simulink model "RefuelSystem"  (R2025a)
settings: Solver=ode23tb  StartTime=0.0  StopTime=1000  MaxStep=0.1  RelTol=1e-3
libraries: simulink x5
settings Model: DataDictionary=FuelGaugingData.sldd  Creator=mkelley  LastModifiedBy=mkelley

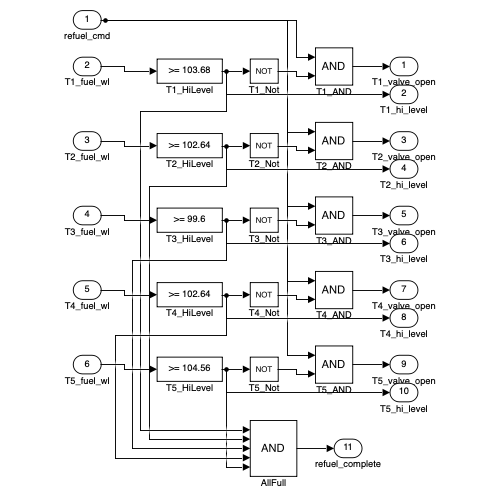
[thumbnail: Simulink's stored preview of the top-level diagram]
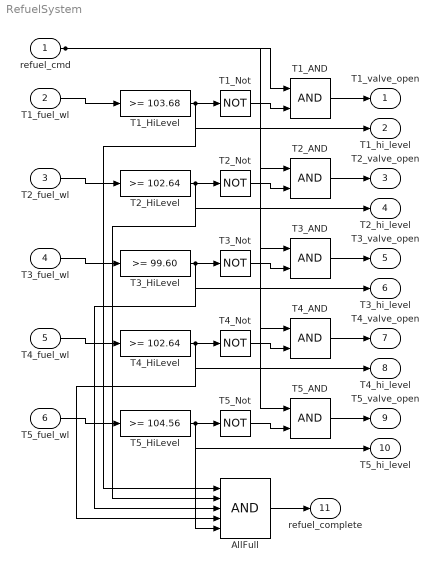
== system RefuelSystem ==
  refuel_cmd : Inport
  T1_fuel_wl : Inport  Port=2
  T2_fuel_wl : Inport  Port=3
  T3_fuel_wl : Inport  Port=4
  T4_fuel_wl : Inport  Port=5
  T5_fuel_wl : Inport  Port=6
  AllFull : Logic  Inputs=5  AllPortsSameDT=off  OutDataTypeStr=boolean
  T1_AND : Logic  AllPortsSameDT=off  OutDataTypeStr=boolean
  T1_HiLevel : simulink/Logic and Bit Operations/Compare To Constant  relop=>=  const=103.68  OutDataTypeStr=boolean
  T1_Not : Logic  Operator=NOT  AllPortsSameDT=off  OutDataTypeStr=boolean
  T2_AND : Logic  AllPortsSameDT=off  OutDataTypeStr=boolean
  T2_HiLevel : simulink/Logic and Bit Operations/Compare To Constant  relop=>=  const=102.64  OutDataTypeStr=boolean
  T2_Not : Logic  Operator=NOT  AllPortsSameDT=off  OutDataTypeStr=boolean
  T3_AND : Logic  AllPortsSameDT=off  OutDataTypeStr=boolean
  T3_HiLevel : simulink/Logic and Bit Operations/Compare To Constant  relop=>=  const=99.60  OutDataTypeStr=boolean
  T3_Not : Logic  Operator=NOT  AllPortsSameDT=off  OutDataTypeStr=boolean
  T4_AND : Logic  AllPortsSameDT=off  OutDataTypeStr=boolean
  T4_HiLevel : simulink/Logic and Bit Operations/Compare To Constant  relop=>=  const=102.64  OutDataTypeStr=boolean
  T4_Not : Logic  Operator=NOT  AllPortsSameDT=off  OutDataTypeStr=boolean
  T5_AND : Logic  AllPortsSameDT=off  OutDataTypeStr=boolean
  T5_HiLevel : simulink/Logic and Bit Operations/Compare To Constant  relop=>=  const=104.56  OutDataTypeStr=boolean
  T5_Not : Logic  Operator=NOT  AllPortsSameDT=off  OutDataTypeStr=boolean
  T1_valve_open : Outport
  T1_hi_level : Outport  Port=2
  T2_valve_open : Outport  Port=3
  T2_hi_level : Outport  Port=4
  T3_valve_open : Outport  Port=5
  T3_hi_level : Outport  Port=6
  T4_valve_open : Outport  Port=7
  T4_hi_level : Outport  Port=8
  T5_valve_open : Outport  Port=9
  T5_hi_level : Outport  Port=10
  refuel_complete : Outport  Port=11
  wires:
  T1_fuel_wl/1 -> T1_HiLevel/1
  T1_HiLevel/1 -> T1_Not/1, T1_hi_level/1, AllFull/1
  refuel_cmd/1 -> T1_AND/1, T2_AND/1, T3_AND/1, T4_AND/1, T5_AND/1
  T1_Not/1 -> T1_AND/2
  T1_AND/1 -> T1_valve_open/1
  T2_fuel_wl/1 -> T2_HiLevel/1
  T2_HiLevel/1 -> T2_Not/1, T2_hi_level/1, AllFull/2
  T2_Not/1 -> T2_AND/2
  T2_AND/1 -> T2_valve_open/1
  T3_fuel_wl/1 -> T3_HiLevel/1
  T3_HiLevel/1 -> T3_Not/1, T3_hi_level/1, AllFull/3
  T3_Not/1 -> T3_AND/2
  T3_AND/1 -> T3_valve_open/1
  T4_fuel_wl/1 -> T4_HiLevel/1
  T4_HiLevel/1 -> T4_Not/1, T4_hi_level/1, AllFull/4
  T4_Not/1 -> T4_AND/2
  T4_AND/1 -> T4_valve_open/1
  T5_fuel_wl/1 -> T5_HiLevel/1
  T5_HiLevel/1 -> T5_Not/1, T5_hi_level/1, AllFull/5
  T5_Not/1 -> T5_AND/2
  T5_AND/1 -> T5_valve_open/1
  AllFull/1 -> refuel_complete/1
